simulink model "Exp7_DM"  (R2026a)
settings: Solver=VariableStepAuto  StopTime=1
settings Model: Creator=yatha  LastModifiedBy=yatha

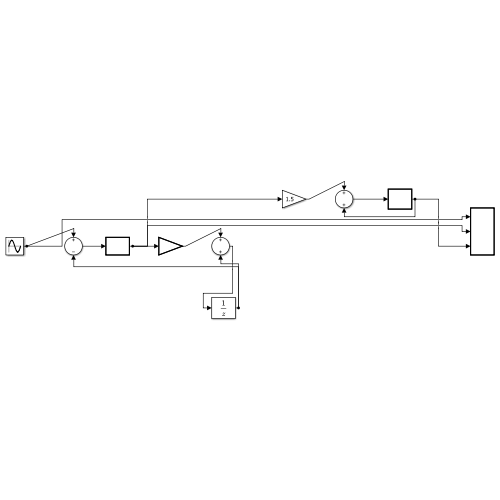
[thumbnail: Simulink's stored preview of the top-level diagram]
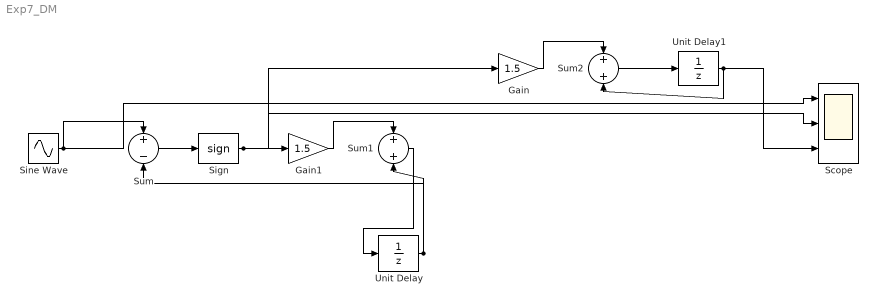
== system Exp7_DM ==
  Gain : Gain  Gain=1.5
  Gain1 : Gain  Gain=1.5
  Scope : Scope  NumInputPorts=3
  Sign : Signum
  Sine Wave : Sin  Amplitude=5  Frequency=12.5664  SampleTime=0
  Sum : Sum  Inputs=+-
  Sum1 : Sum
  Sum2 : Sum
  Unit Delay : UnitDelay  SampleTime=0.05
  Unit Delay1 : UnitDelay  SampleTime=0.05
  wires:
  Sine Wave/1 -> Sum/1, Scope/1
  Sum/1 -> Sign/1
  Sign/1 -> Gain1/1, Gain/1, Scope/2
  Gain1/1 -> Sum1/1
  Sum1/1 -> Unit Delay/1
  Unit Delay/1 -> Sum1/2, Sum/2
  Gain/1 -> Sum2/1
  Sum2/1 -> Unit Delay1/1
  Unit Delay1/1 -> Sum2/2, Scope/3
